simulink model "aAdaptivesInveresFilter_2021b_"  (R2024b)
settings: Solver=ode45  StartTime=0.0  StopTime=10000.0  RelTol=1e-3  EnableMultiTasking=on
undefined symbols (not defined in the file): Amplitudengang, Koeffizienten, LMS, RLS
libraries: dspadpt3 x2, dspspect3 x2, simulink x2
settings Model: Creator=Wirnitzer  LastModifiedBy=49179
settings SolverCC: AlgebraicLoopSolver=TrustRegion
settings DataIOCC: LimitDataPoints=on  SaveFormat=Array  SignalLoggingSaveFormat=ModelDataLogs  ReturnWorkspaceOutputs=off
settings OptimizationCC: BooleanDataType=off  InitFltsAndDblsToZero=on  LifeSpan=inf
settings DebuggingCC: SaveWithParameterizedLinksMsg=none  UnderspecifiedInitializationDetection=Classic  MergeDetectMultiDrivingBlocksExec=none  SignalResolutionControl=TryResolveAllWithWarning  MultiTaskDSMMsg=warning  MultiTaskCondExecSysMsg=none  FcnCallInpInsideContextMsg=warning  UnconnectedInputMsg=warning  UnconnectedOutputMsg=warning  UnconnectedLineMsg=warning  SFUnexpectedBacktrackingDiag=warning  SFNoUnconditionalDefaultTransitionDiag=warning  SFExecutionAtInitializationDiag=none  ArithmeticOperatorsInVariantConditions=warning
settings HardwareCC: ProdBitPerPointer=32  ProdBitPerSizeT=32  ProdBitPerPtrDiffT=32  ProdLargestAtomicFloat=None  ProdIntDivRoundTo=Undefined  ProdEndianess=Unspecified  ProdWordSize=32  ProdHWDeviceType=32-bit Generic  TargetUnknown=on
settings ModelReferenceCC: EnableRefExpFcnMdlSchedulingChecks=on  PropagateSignalLabelsOutOfModel=off
settings RTWCC: GPUComputeCapability=3.5  DLArmComputeVersion=19.05
settings CodeAppCC: StateflowObjectComments=on
settings GRTTargetCC: TargetFcnLib=ansi_tfl_tmw.mat  TargetLangStandard=C89/C90 (ANSI)  ModelReferenceCompliant=off  CombineOutputUpdateFcns=off  MatFileLogging=off  GRTInterface=on
settings ConfigComp: CovMetricSettings=dw  CovSaveCumulativeToWorkspaceVar=on  CovSaveSingleToWorkspaceVar=on

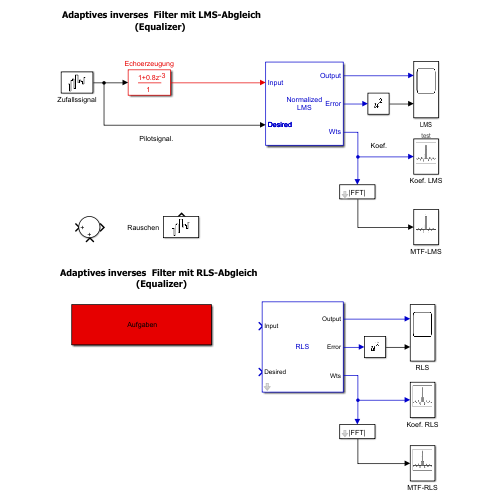
[thumbnail: Simulink's stored preview of the top-level diagram]
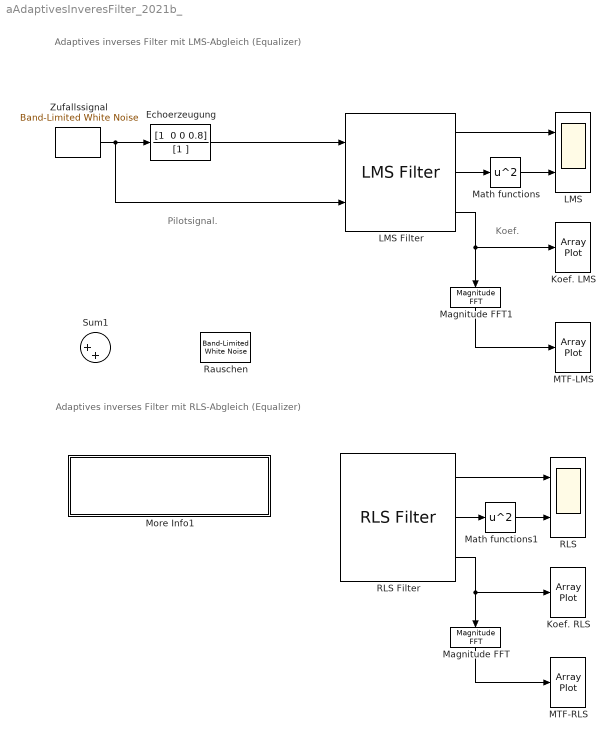
== system aAdaptivesInveresFilter_2021b_ ==
  note: Pilotsignal.
  note: Adaptives inverses  Filter mit RLS-Abgleich
      |  (Equalizer)
  note: Koef.
  note: Adaptives inverses  Filter mit LMS-Abgleich
      | (Equalizer)
  Echoerzeugung : DiscreteFilter  Numerator="[1  0 0 0.8]"  Denominator=[1 ]  SampleTime=1
  Koef. LMS : ArrayPlot  WindowPosition=[285.000000,21.000000,800.000000,500.000000,]  ScopeFrameLocation=window  AxesScaling=Manual  XLabel=Index  YLabel=LMS-Koeffizienten  DefaultConfigurationName=dsp.scopes.ArrayPlotBlockSpecification
  Koef. RLS : ArrayPlot  WindowPosition=[240.000000,110.000000,800.000000,500.000000,]  ScopeFrameLocation=window  AxesScaling=Manual  XLabel=Index  YLabel=RLS-Koeffizienten  DefaultConfigurationName=dsp.scopes.ArrayPlotBlockSpecification
  LMS : Scope  NumInputPorts=2
      settings: AttributesFormatString=test
  LMS Filter : dspadpt3/LMS Filter  Algo=Normalized LMS  L=11  stepflag=Dialog  mu=0.05  leakage=1.0  ic=0  Adapt=off  resetflag=None  weights=on  addnparflag=off  roundingMode=Floor  overflowMode=off  secondCoeffMode=Binary point scaling  secondCoeffWordLength=2  secondCoeffFracLength=15  prodOutput2Mode=Binary point scaling  prodOutput2FracLength=20  prodOutput3Mode=Binary point scaling  prodOutput3FracLength=20  prodOutput4Mode=Binary point scaling  prodOutput4FracLength=20  quotientMode=Binary point scaling  quotientFracLength=20  accum2Mode=Binary point scaling  accum2FracLength=20
  MTF-LMS : ArrayPlot  WindowPosition=[153.000000,27.000000,801.000000,500.000000,]  ScopeFrameLocation=window  AxesScaling=Manual  XLabel=Frequenzzahl  YLabel=LMS-Amplitudengang  DefaultConfigurationName=dsp.scopes.ArrayPlotBlockSpecification
  MTF-RLS : ArrayPlot  WindowPosition=[240.000000,110.000000,800.000000,500.000000,]  ScopeFrameLocation=window  AxesScaling=Manual  XLabel=Frequenzzahl  YLabel=RLS-Amplitudengang  DefaultConfigurationName=dsp.scopes.ArrayPlotBlockSpecification
  Magnitude FFT : dspspect3/Magnitude FFT  mag_or_magsq=Magnitude  FFTImplementation=Auto  fftLenInherit=off  fftsize=256  WrapInput=on
  Magnitude FFT1 : dspspect3/Magnitude FFT  mag_or_magsq=Magnitude  FFTImplementation=Auto  fftLenInherit=off  fftsize=256  WrapInput=on
  Math functions : Math  Operator=square  SignedPower=on
  Math functions1 : Math  Operator=square  SignedPower=on
  More Info1 : Subsystem
      mask Display: disp(' Aufgaben')
  RLS : Scope  NumInputPorts=2
  RLS Filter : dspadpt3/RLS Filter  L=11  lambdaflag=Dialog  lambda=0.999  addnparflag=on  ic=0  delta=0.1  Adapt=off  resetflag=None  weights=on
  Rauschen : simulink/Sources/Band-Limited White Noise  Cov=0.3  Ts=1  seed=[241]
  Sum1 : Sum  Inputs=|++  InputSameDT=on  SaturateOnIntegerOverflow=on  OutDataTypeStr=Inherit: Same as first input
  Zufallssignal : simulink/Sources/Band-Limited White Noise  Cov=1  Ts=1  seed=[23341]
  wires:
  Math functions/1 -> LMS/2
  LMS Filter/1 -> LMS/1
  LMS Filter/2 -> Math functions/1
  LMS Filter/3 -> Koef. LMS/1, Magnitude FFT1/1
  Zufallssignal/1 -> Echoerzeugung/1, LMS Filter/2
  Math functions1/1 -> RLS/2
  RLS Filter/1 -> RLS/1
  RLS Filter/2 -> Math functions1/1
  RLS Filter/3 -> Koef. RLS/1, Magnitude FFT/1
  Magnitude FFT/1 -> MTF-RLS/1
  Magnitude FFT1/1 -> MTF-LMS/1
  Echoerzeugung/1 -> LMS Filter/1

== system aAdaptivesInveresFilter_2021b_/More Info1 ==
  note: Adaptives Inverses System (== Entzerrer == Equalizer)
      | ===========================================
      | (c) HSM, B. Wir 7.11 97, 8.8.2012
      |
      |
      | Starten Sie die Simulation mit  SIMULATION, START.
      | Beobachten Sie wie sich die Koeffizienten des Filters langsam einstellen.
      | Durch einen Doppelklick auf das Oszilloskop können Sie die Signale
      | beobachten. Mit der rechten Maustate können Sie AUTOSCALE aktivieren.
      |
      | (i)   Stellen sich die erwarteten Filterkoeffizienten ein?
      |
      | (ii)  Welche Einflüsse haben die Filterordnung und die Schrittweite des LMS auf das Ergebnis?
      |
      | (iii) Addieren Sie Rauschen zum System und untersuchen Sie (i) und (ii).
      |
      | (iv) Welche Vorteile bringt der RLS-Algorithmus?
      |
      | (v)  Entzerren Sie den Übertragungskanal \( G(z) = 1 + 2z^{-1} + z^{-3} \) und beantworten Sie (i)-(iv).
